simulink model "adptive"  (R2017b)
settings: Solver=VariableStepAuto  StartTime=0.0  StopTime=10  RelTol=1e-3
PreLoadFcn:
  | init.m;
libraries: simulink x2
settings Model: Creator=Administrator  LastModifiedBy=Administrator
settings SolverCC: ZeroCrossAlgorithm=Adaptive
settings DebuggingCC: MaxConsecutiveZCsMsg=none

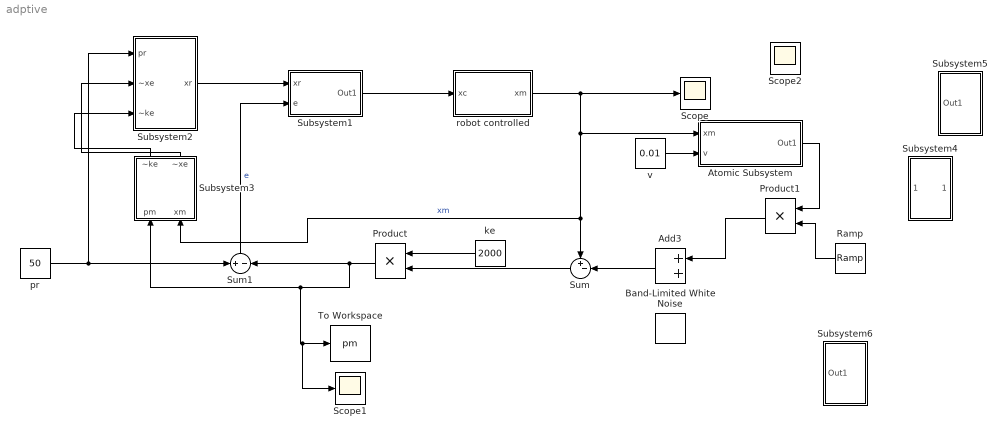
== system adptive ==
  Add3 : Sum
  Atomic Subsystem : Subsystem  TreatAsAtomicUnit=on
  Band-Limited White Noise : simulink/Sources/Band-Limited White Noise  Cov=[0.000000001]  Ts=0.01  seed=[23341]
  Product : Product
  Product1 : Product
  Ramp : simulink/Sources/Ramp  slope=0.5  start=0  X0=1
  Scope : Scope
  Scope1 : Scope
  Scope2 : Scope
  Subsystem1 : Subsystem
  Subsystem2 : Subsystem
  Subsystem3 : Subsystem
  Subsystem4 : Subsystem
  Subsystem5 : Subsystem
  Subsystem6 : Subsystem
  Sum : Sum  Inputs=+-|
  Sum1 : Sum  Inputs=+|-
  To Workspace : ToWorkspace  VariableName=pm  SaveFormat=Timeseries  SampleTime=-1
  ke : Constant  Value=2000
  pr : Constant  Value=50
  robot controlled : Subsystem
  v : Constant  Value=0.01
  wires:
  Subsystem3/1(~ke) -> Subsystem2/3(~ke)
  pr/1 -> Subsystem2/1(pr), Sum1/1
  Subsystem3/2(~xe) -> Subsystem2/2(~xe)
  Sum1/1 -> Subsystem1/2(e)  "e"
  Subsystem2/1(xr) -> Subsystem1/1(xr)
  Product/1 -> Scope1/1, To Workspace/1, Subsystem3/1(pm), Sum1/2
  Sum/1 -> Product/2
  robot controlled/1("xm ") -> Atomic Subsystem/1(xm), Subsystem3/2(xm), Sum/1, Scope/1  "xm"
  ke/1 -> Product/1
  Add3/1 -> Sum/2
  Subsystem1/1(Out1) -> robot controlled/1(xc)
  v/1 -> Atomic Subsystem/2(v)
  Atomic Subsystem/1(Out1) -> Product1/1
  Ramp/1 -> Product1/2
  Product1/1 -> Add3/1

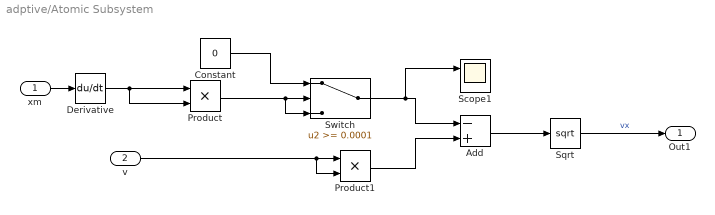
== system adptive/Atomic Subsystem ==
  xm : Inport
  v : Inport  Port=2
  Add : Sum  Inputs=-+
  Constant : Constant  Value=0
  Derivative : Derivative
  Product : Product
  Product1 : Product
  Scope1 : Scope  NumInputPorts=2
  Sqrt : Sqrt  SaturateOnIntegerOverflow=on
  Switch : Switch  Threshold=0.0001
  Out1 : Outport
  wires:
  xm/1 -> Derivative/1
  v/1 -> Product1/2, Product1/1
  Product1/1 -> Add/2
  Add/1 -> Sqrt/1
  Sqrt/1 -> Out1/1  "vx"
  Derivative/1 -> Product/2, Product/1
  Switch/1 -> Scope1/1, Add/1
  Constant/1 -> Switch/1
  Product/1 -> Switch/3, Switch/2

== system adptive/Subsystem1 ==
  xr : Inport
  e : Inport  Port=2
  Add : Sum
  Gain : Gain  Gain=5000
  Transfer Fcn : TransferFcn  Denominator=[1 800 5000]
  Out1 : Outport
  wires:
  xr/1 -> Gain/1
  Gain/1 -> Add/1
  e/1 -> Add/2
  Add/1 -> Transfer Fcn/1
  Transfer Fcn/1 -> Out1/1

== system adptive/Subsystem2 ==
  note: ~xe
  note: ~ke
  pr : Inport
  ~xe : Inport  Port=2
  ~ke : Inport  Port=3
  Add : Sum
  Divide : Product  Inputs=*/
  xr : Outport
  wires:
  pr/1 -> Divide/1
  ~ke/1 -> Divide/2
  ~xe/1 -> Add/1
  Divide/1 -> Add/2
  Add/1 -> xr/1

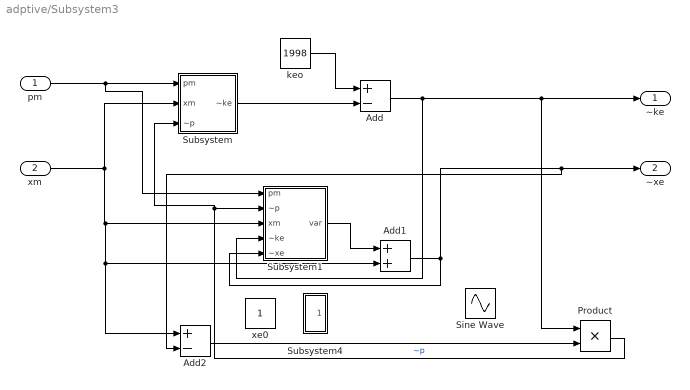
== system adptive/Subsystem3 ==
  pm : Inport
  xm : Inport  Port=2
  Add : Sum  Inputs=+-
  Add1 : Sum
  Add2 : Sum  Inputs=+-
  Product : Product
  Sine Wave : Sin  SampleTime=0
  Subsystem : Subsystem
  Subsystem1 : Subsystem
  Subsystem4 : Subsystem
  keo : Constant  Value=1998
  xe0 : Constant
  ~ke : Outport
  ~xe : Outport  Port=2
  wires:
  pm/1 -> Subsystem1/1(pm), Subsystem/1(pm)
  xm/1 -> Subsystem/2(xm), Add1/2, Add2/1, Subsystem1/3(xm)
  Add/1 -> Subsystem1/4(~ke), Product/1, ~ke/1
  Subsystem/1(~ke) -> Add/2
  Subsystem1/1(var) -> Add1/1
  Add1/1 -> Subsystem1/5("~xe "), Add2/2, ~xe/1
  Add2/1 -> Product/2
  Product/1 -> Subsystem/3(~p), Subsystem1/2(~p)  "~p"
  keo/1 -> Add/1

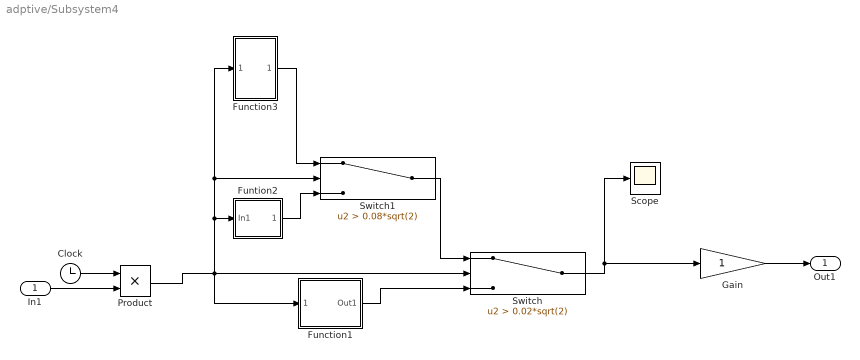
== system adptive/Subsystem4 ==
  In1 : Inport
  Clock : Clock
  Function1 : Subsystem
  Function3 : Subsystem
  Funtion2 : Subsystem
  Gain : Gain
  Product : Product
  Scope : Scope
  Switch : Switch  Criteria=u2 > Threshold  Threshold=0.02*sqrt(2)
  Switch1 : Switch  Criteria=u2 > Threshold  Threshold=0.08*sqrt(2)
  Out1 : Outport
  wires:
  Function3/1(Out1) -> Switch1/1
  Funtion2/1(Out1) -> Switch1/3
  Clock/1 -> Product/1
  Product/1 -> Function1/1(time in), Switch/2, Function3/1(In1), Switch1/2, Funtion2/1(In1)
  Switch1/1 -> Switch/1
  Switch/1 -> Gain/1, Scope/1
  Function1/1(Out1) -> Switch/3
  Gain/1 -> Out1/1
  In1/1 -> Product/2

== system adptive/Subsystem5 ==
  Clock : Clock
  Function1 : Subsystem
  Function3 : Subsystem
  Funtion2 : Subsystem
  Gain : Gain
  Gain1 : Gain  Gain=1/1000
  Scope : Scope
  Switch : Switch  Criteria=u2 > Threshold  Threshold=0.0282842712474619
  Switch1 : Switch  Criteria=u2 > Threshold  Threshold=0.1131370849898476
  Out1 : Outport
  wires:
  Gain/1 -> Out1/1
  Function1/1(Out1) -> Switch/3
  Switch/1 -> Scope/1, Gain/1
  Switch1/1 -> Switch/1
  Clock/1 -> Gain1/1
  Funtion2/1(Out1) -> Switch1/3
  Function3/1(Out1) -> Switch1/1
  Gain1/1 -> Funtion2/1(In1), Switch1/2, Function3/1(In1), Switch/2, Function1/1(time in)

== system adptive/Subsystem6 ==
  Clock : Clock
  Function1 : Subsystem
  Function3 : Subsystem
  Funtion2 : Subsystem
  Gain : Gain
  Gain1 : Gain  Gain=5/1000
  Scope : Scope
  Switch : Switch  Criteria=u2 > Threshold  Threshold=0.02*sqrt(2)
  Switch1 : Switch  Criteria=u2 > Threshold  Threshold=0.08*sqrt(2)
  Out1 : Outport
  wires:
  Gain/1 -> Out1/1
  Function1/1(Out1) -> Switch/3
  Switch/1 -> Scope/1, Gain/1
  Switch1/1 -> Switch/1
  Clock/1 -> Gain1/1
  Funtion2/1(Out1) -> Switch1/3
  Function3/1(Out1) -> Switch1/1
  Gain1/1 -> Funtion2/1(In1), Switch1/2, Function3/1(In1), Switch/2, Function1/1(time in)

== system adptive/robot controlled ==
  xc : Inport
  Switch : Switch  Criteria=u2 ~= 0  Threshold=0.1
  "xm " : Outport
  wires:
  xc/1 -> "xm "/1

== system adptive/Subsystem3/Subsystem ==
  pm : Inport
  xm : Inport  Port=2
  ~p : Inport  Port=3
  Add : Sum  Inputs=-+
  Integrator : Integrator
  Product : Product
  Product1 : Product
  Subsystem1 : Subsystem
  ~ke : Outport
  wires:
  ~p/1 -> Add/2
  pm/1 -> Add/1
  xm/1 -> Product/1
  Add/1 -> Product/2
  Product/1 -> Integrator/1
  Integrator/1 -> Product1/2
  Product1/1 -> ~ke/1
  Subsystem1/1(γ1) -> Product1/1

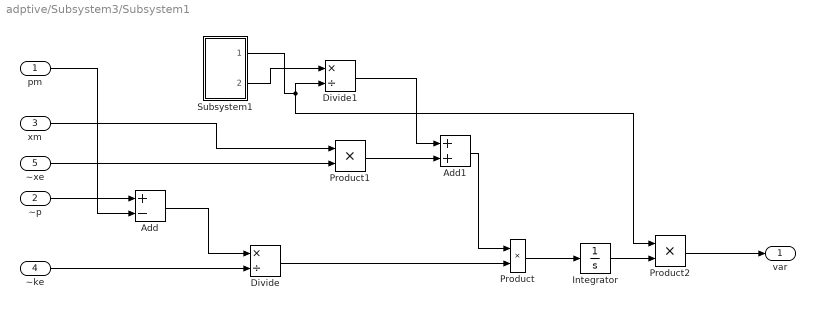
== system adptive/Subsystem3/Subsystem1 ==
  pm : Inport
  ~p : Inport  Port=2
  xm : Inport  Port=3
  ~ke : Inport  Port=4
  "~xe " : Inport  Port=5
  Add : Sum  Inputs=+-
  Add1 : Sum
  Divide : Product  Inputs=*/
  Divide1 : Product  Inputs=*/
  Integrator : Integrator
  Product : Product
  Product1 : Product
  Product2 : Product
  Subsystem1 : Subsystem
  var : Outport
  wires:
  pm/1 -> Add/2
  ~p/1 -> Add/1
  Add/1 -> Divide/1
  ~ke/1 -> Divide/2
  Divide/1 -> Product/2
  xm/1 -> Product1/1
  Divide1/1 -> Add1/1
  Product1/1 -> Add1/2
  Add1/1 -> Product/1
  Integrator/1 -> Product2/2
  Product2/1 -> var/1
  "~xe "/1 -> Product1/2
  Product/1 -> Integrator/1
  Subsystem1/2(gama2) -> Divide1/1
  Subsystem1/1(gama1) -> Product2/1, Divide1/2

== system adptive/Subsystem3/Subsystem4 ==
  Clock : Clock
  Function1 : Subsystem
  Function3 : Subsystem
  Funtion2 : Subsystem
  Gain : Gain  Gain=1/1000
  Scope : Scope
  Switch : Switch  Criteria=u2 > Threshold  Threshold=28.2842712474619
  Switch1 : Switch  Criteria=u2 > Threshold  Threshold=113.1370849898476
  Velocity : Gain  Gain=5
  Out1 : Outport
  wires:
  Function3/1(Out1) -> Switch1/1
  Funtion2/1(Out1) -> Switch1/3
  Clock/1 -> Velocity/1
  Velocity/1 -> Function1/1(time in), Switch/2, Function3/1(In1), Switch1/2, Funtion2/1(In1)
  Switch1/1 -> Switch/1
  Switch/1 -> Gain/1, Scope/1
  Function1/1(Out1) -> Switch/3
  Gain/1 -> Out1/1

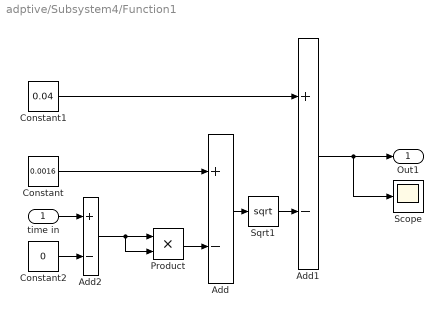
== system adptive/Subsystem4/Function1 ==
  time in : Inport
  Add : Sum  Inputs=+-
  Add1 : Sum  Inputs=+-
  Add2 : Sum  Inputs=+-
  Constant : Constant  Value=0.0016
  Constant1 : Constant  Value=0.04
  Constant2 : Constant  Value=0
  Product : Product
  Scope : Scope
  Sqrt1 : Sqrt  SaturateOnIntegerOverflow=on
  Out1 : Outport
  wires:
  Constant/1 -> Add/1
  time in/1 -> Add2/1
  Constant2/1 -> Add2/2
  Add2/1 -> Product/2, Product/1
  Product/1 -> Add/2
  Add/1 -> Sqrt1/1
  Sqrt1/1 -> Add1/2
  Constant1/1 -> Add1/1
  Add1/1 -> Out1/1, Scope/1

== system adptive/Subsystem4/Function3 ==
  In1 : Inport
  Add : Sum  Inputs=+-
  Add1 : Sum  Inputs=+-
  Add2 : Sum  Inputs=+-
  Product1 : Product
  Sqrt : Sqrt  SaturateOnIntegerOverflow=on
  pr2 : Constant  Value=0.0016
  pr3 : Constant  Value=0.1*sqrt(2)
  pr4 : Constant  Value=0.04
  Out1 : Outport
  wires:
  Add2/1 -> Out1/1
  pr3/1 -> Add1/2
  In1/1 -> Add1/1
  Add1/1 -> Product1/2, Product1/1
  Product1/1 -> Add/2
  pr2/1 -> Add/1
  Add/1 -> Sqrt/1
  pr4/1 -> Add2/1
  Sqrt/1 -> Add2/2

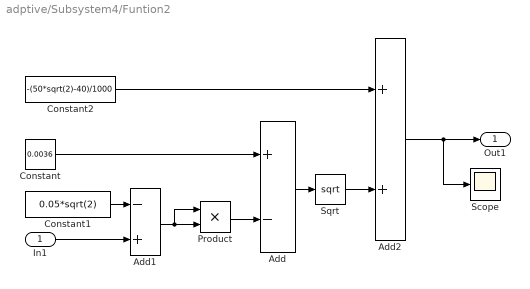
== system adptive/Subsystem4/Funtion2 ==
  In1 : Inport
  Add : Sum  Inputs=+-
  Add1 : Sum  Inputs=-+
  Add2 : Sum
  Constant : Constant  Value=0.0036
  Constant1 : Constant  Value=0.05*sqrt(2)
  Constant2 : Constant  Value=-(50*sqrt(2)-40)/1000
  Product : Product
  Scope : Scope
  Sqrt : Sqrt  SaturateOnIntegerOverflow=on
  Out1 : Outport
  wires:
  Constant/1 -> Add/1
  In1/1 -> Add1/2
  Add1/1 -> Product/1, Product/2
  Product/1 -> Add/2
  Constant1/1 -> Add1/1
  Add/1 -> Sqrt/1
  Sqrt/1 -> Add2/2
  Constant2/1 -> Add2/1
  Add2/1 -> Scope/1, Out1/1

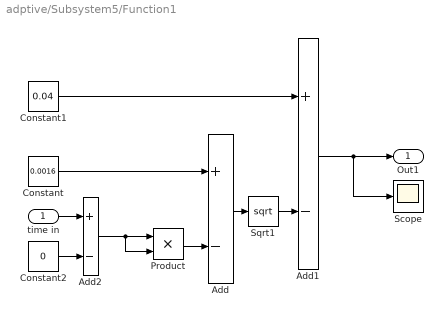
== system adptive/Subsystem5/Function1 ==
  time in : Inport
  Add : Sum  Inputs=+-
  Add1 : Sum  Inputs=+-
  Add2 : Sum  Inputs=+-
  Constant : Constant  Value=0.0016
  Constant1 : Constant  Value=0.04
  Constant2 : Constant  Value=0
  Product : Product
  Scope : Scope
  Sqrt1 : Sqrt  SaturateOnIntegerOverflow=on
  Out1 : Outport
  wires:
  Add1/1 -> Scope/1, Out1/1
  Constant1/1 -> Add1/1
  Sqrt1/1 -> Add1/2
  Add/1 -> Sqrt1/1
  Product/1 -> Add/2
  Add2/1 -> Product/1, Product/2
  Constant2/1 -> Add2/2
  time in/1 -> Add2/1
  Constant/1 -> Add/1

== system adptive/Subsystem5/Function3 ==
  In1 : Inport
  Add : Sum  Inputs=+-
  Add1 : Sum  Inputs=+-
  Add2 : Sum  Inputs=+-
  Product1 : Product
  Sqrt : Sqrt  SaturateOnIntegerOverflow=on
  pr2 : Constant  Value=0.0016
  pr3 : Constant  Value=0.14142135623731
  pr4 : Constant  Value=0.04
  Out1 : Outport
  wires:
  Sqrt/1 -> Add2/2
  pr4/1 -> Add2/1
  Add/1 -> Sqrt/1
  pr2/1 -> Add/1
  Product1/1 -> Add/2
  Add1/1 -> Product1/1, Product1/2
  In1/1 -> Add1/1
  pr3/1 -> Add1/2
  Add2/1 -> Out1/1

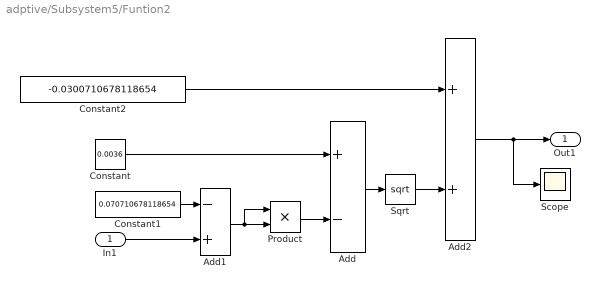
== system adptive/Subsystem5/Funtion2 ==
  In1 : Inport
  Add : Sum  Inputs=+-
  Add1 : Sum  Inputs=-+
  Add2 : Sum
  Constant : Constant  Value=0.0036
  Constant1 : Constant  Value=0.070710678118654
  Constant2 : Constant  Value=-0.0300710678118654
  Product : Product
  Scope : Scope
  Sqrt : Sqrt  SaturateOnIntegerOverflow=on
  Out1 : Outport
  wires:
  Add2/1 -> Out1/1, Scope/1
  Constant2/1 -> Add2/1
  Sqrt/1 -> Add2/2
  Add/1 -> Sqrt/1
  Constant1/1 -> Add1/1
  Product/1 -> Add/2
  Add1/1 -> Product/2, Product/1
  In1/1 -> Add1/2
  Constant/1 -> Add/1

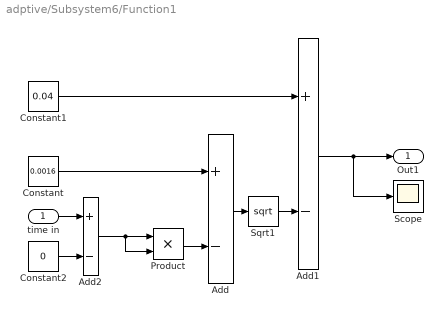
== system adptive/Subsystem6/Function1 ==
  time in : Inport
  Add : Sum  Inputs=+-
  Add1 : Sum  Inputs=+-
  Add2 : Sum  Inputs=+-
  Constant : Constant  Value=0.0016
  Constant1 : Constant  Value=0.04
  Constant2 : Constant  Value=0
  Product : Product
  Scope : Scope
  Sqrt1 : Sqrt  SaturateOnIntegerOverflow=on
  Out1 : Outport
  wires:
  Add1/1 -> Scope/1, Out1/1
  Constant1/1 -> Add1/1
  Sqrt1/1 -> Add1/2
  Add/1 -> Sqrt1/1
  Product/1 -> Add/2
  Add2/1 -> Product/1, Product/2
  Constant2/1 -> Add2/2
  time in/1 -> Add2/1
  Constant/1 -> Add/1

== system adptive/Subsystem6/Function3 ==
  In1 : Inport
  Add : Sum  Inputs=+-
  Add1 : Sum  Inputs=+-
  Add2 : Sum  Inputs=+-
  Product1 : Product
  Sqrt : Sqrt  SaturateOnIntegerOverflow=on
  pr2 : Constant  Value=0.0016
  pr3 : Constant  Value=0.1*sqrt(2)
  pr4 : Constant  Value=0.04
  Out1 : Outport
  wires:
  Sqrt/1 -> Add2/2
  pr4/1 -> Add2/1
  Add/1 -> Sqrt/1
  pr2/1 -> Add/1
  Product1/1 -> Add/2
  Add1/1 -> Product1/1, Product1/2
  In1/1 -> Add1/1
  pr3/1 -> Add1/2
  Add2/1 -> Out1/1

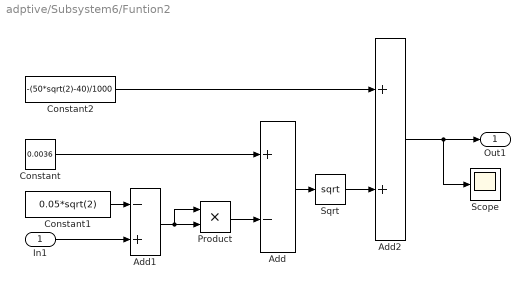
== system adptive/Subsystem6/Funtion2 ==
  In1 : Inport
  Add : Sum  Inputs=+-
  Add1 : Sum  Inputs=-+
  Add2 : Sum
  Constant : Constant  Value=0.0036
  Constant1 : Constant  Value=0.05*sqrt(2)
  Constant2 : Constant  Value=-(50*sqrt(2)-40)/1000
  Product : Product
  Scope : Scope
  Sqrt : Sqrt  SaturateOnIntegerOverflow=on
  Out1 : Outport
  wires:
  Add2/1 -> Out1/1, Scope/1
  Constant2/1 -> Add2/1
  Sqrt/1 -> Add2/2
  Add/1 -> Sqrt/1
  Constant1/1 -> Add1/1
  Product/1 -> Add/2
  Add1/1 -> Product/2, Product/1
  In1/1 -> Add1/2
  Constant/1 -> Add/1

== system adptive/Subsystem3/Subsystem/Subsystem1 ==
  Demux : Demux  Outputs=2
  From Workspace : FromWorkspace  VariableName=simin  SampleTime=0
  Scope : Scope
  γ1 : Outport
  γ2 : Outport  Port=2
  wires:
  Demux/2 -> γ2/1
  Demux/1 -> γ1/1
  From Workspace/1 -> Scope/1, Demux/1

== system adptive/Subsystem3/Subsystem1/Subsystem1 ==
  Demux : Demux  Outputs=2
  From Workspace : FromWorkspace  VariableName=simin  SampleTime=0
  Scope : Scope
  gama1 : Outport
  gama2 : Outport  Port=2
  wires:
  Demux/2 -> gama2/1
  Demux/1 -> Scope/1, gama1/1
  From Workspace/1 -> Demux/1

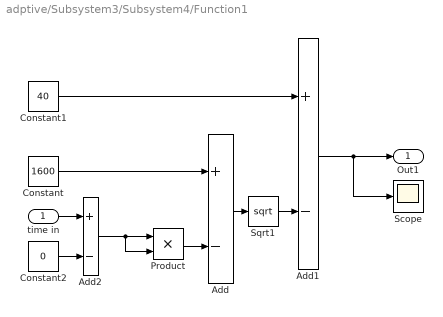
== system adptive/Subsystem3/Subsystem4/Function1 ==
  time in : Inport
  Add : Sum  Inputs=+-
  Add1 : Sum  Inputs=+-
  Add2 : Sum  Inputs=+-
  Constant : Constant  Value=1600
  Constant1 : Constant  Value=40
  Constant2 : Constant  Value=0
  Product : Product
  Scope : Scope
  Sqrt1 : Sqrt  SaturateOnIntegerOverflow=on
  Out1 : Outport
  wires:
  Constant/1 -> Add/1
  time in/1 -> Add2/1
  Constant2/1 -> Add2/2
  Add2/1 -> Product/2, Product/1
  Product/1 -> Add/2
  Add/1 -> Sqrt1/1
  Sqrt1/1 -> Add1/2
  Constant1/1 -> Add1/1
  Add1/1 -> Out1/1, Scope/1

== system adptive/Subsystem3/Subsystem4/Function3 ==
  In1 : Inport
  Add : Sum  Inputs=+-
  Add1 : Sum  Inputs=+-
  Add2 : Sum  Inputs=+-
  Product1 : Product
  Sqrt : Sqrt  SaturateOnIntegerOverflow=on
  pr2 : Constant  Value=1600
  pr3 : Constant  Value=141.42135623731
  pr4 : Constant  Value=40
  Out1 : Outport
  wires:
  Add2/1 -> Out1/1
  pr3/1 -> Add1/2
  In1/1 -> Add1/1
  Add1/1 -> Product1/2, Product1/1
  Product1/1 -> Add/2
  pr2/1 -> Add/1
  Add/1 -> Sqrt/1
  pr4/1 -> Add2/1
  Sqrt/1 -> Add2/2

== system adptive/Subsystem3/Subsystem4/Funtion2 ==
  In1 : Inport
  Add : Sum  Inputs=+-
  Add1 : Sum  Inputs=-+
  Add2 : Sum
  Constant : Constant  Value=3600
  Constant1 : Constant  Value=70.710678118654
  Constant2 : Constant  Value=-30.710678118654
  Product : Product
  Scope : Scope
  Sqrt : Sqrt  SaturateOnIntegerOverflow=on
  Out1 : Outport
  wires:
  Constant/1 -> Add/1
  In1/1 -> Add1/2
  Add1/1 -> Product/1, Product/2
  Product/1 -> Add/2
  Constant1/1 -> Add1/1
  Add/1 -> Sqrt/1
  Sqrt/1 -> Add2/2
  Constant2/1 -> Add2/1
  Add2/1 -> Scope/1, Out1/1
